simulink library "VrepLib"  (R2021a)
settings: Solver=VariableStepAuto  StartTime=0.0  StopTime=10.0  RelTol=1e-3
values from neighbouring files (symbols this model uses):
  clientID = vrep.simxStart('127.0.0.1', port, true, true, 5000, 5)    [InitSim.m]
  vrep = remApi('remoteApi')    [InitSim.m]
libraries: JointLib x2
settings Model: Creator=Harry  LastModifiedBy=Harry

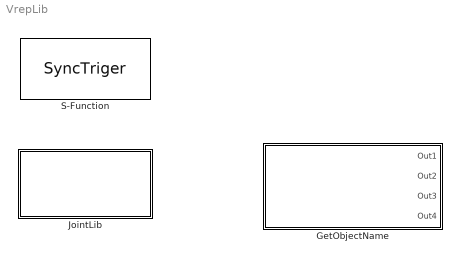
== system VrepLib ==
  GetObjectName : Subsystem  mask{object_name='L1', relative_object_name='world'}
      mask prompts: object_name "Object name:"; relative_object_name "Relative name:"
      mask DialogControl DescGroupVar Prompt: Instructions
      mask DialogControl DescTextVar Prompt: Relative Object: 'world' means relative to world frame, 'parent' means  relative to parent frame, and you can input other object name.
      mask Display:
      | port_label('output',1,'vector(x,y,z)')
      | port_label('output',2,'x')
      | port_label('output',3,'y')
      | port_label('output',4,'z')
      | 
      | if ischar(object_name)
      |     color('black');
      |     x=sprintf('GetObjectName\n%s',object_name);
      |     disp(x);
      | else
      |     color('red');
      |     disp('Input Error');
      | end
  JointLib : Subsystem
      mask Display: image('$imagefile'); % Use "Edit Image" on toolstrip to change.
  S-Function : S-Function  FunctionName=SyncTriger  Parameters=vrep,clientID  SFunctionDeploymentMode=off  EnableBusSupport=off
      mask Display:
      | disp('Sync triger');
      | 
      | 
      | color('red')
      | text(5,8,'VrepSim V0.1')

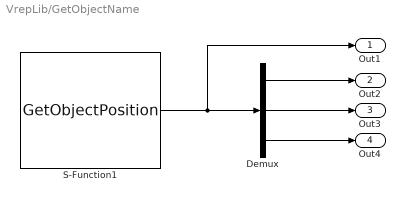
== system VrepLib/GetObjectName ==
  Demux : Demux  Outputs=3
  S-Function1 : S-Function  FunctionName=GetObjectPosition  Parameters=vrep,clientID,object_name,relative_object_name  SFunctionDeploymentMode=off  EnableBusSupport=off
  Out1 : Outport
  Out2 : Outport  Port=2
  Out3 : Outport  Port=3
  Out4 : Outport  Port=4
  wires:
  S-Function1/1 -> Out1/1, Demux/1
  Demux/1 -> Out2/1
  Demux/3 -> Out4/1
  Demux/2 -> Out3/1

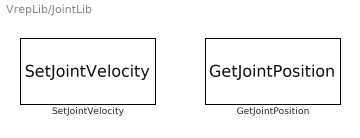
== system VrepLib/JointLib ==
  GetJointPosition : JointLib/GetJointPosition  joint_name='Revolute_joint1'  is_use_radian=off
  SetJointVelocity : JointLib/SetJointVelocity  joint_name='Revolute_joint1'  is_use_radian=on
